simulink model "q3_bilinear"  (R2017b)
settings: Solver=VariableStepAuto  StartTime=0.0  StopTime=5  RelTol=1e-3
settings Model: Creator=admin  LastModifiedBy=admin

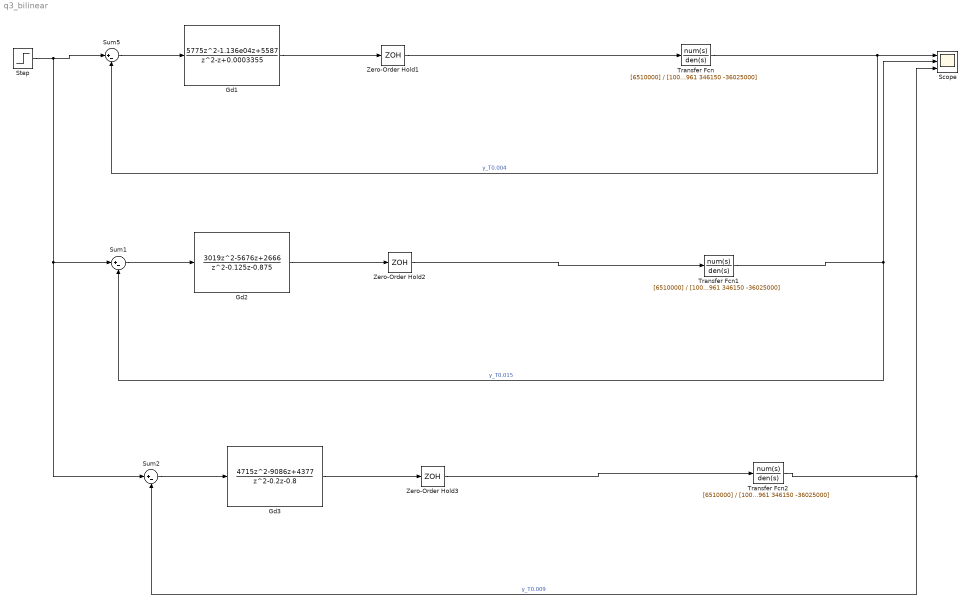
== system q3_bilinear ==
  " Gd1" : DiscreteTransferFcn  Numerator=[5775 -1.136e04 5587]  Denominator=[1 -1 0.0003355]  SampleTime=0.004
  " Gd2" : DiscreteTransferFcn  Numerator=[3019 -5676 2666]  Denominator=[1 -0.125 -0.875]  SampleTime=0.015
  " Gd3" : DiscreteTransferFcn  Numerator=[4715 -9086 4377]  Denominator=[1 -0.2 -0.8]  SampleTime=0.009
  Scope : Scope  NumInputPorts=3
  Step : Step  SampleTime=0
  Sum1 : Sum  Inputs=|+-
  Sum2 : Sum  Inputs=|+-
  Sum5 : Sum  Inputs=|+-
  Transfer Fcn : TransferFcn  Numerator=[6510000]  Denominator=[10000 2501961 346150 -36025000]
  Transfer Fcn1 : TransferFcn  Numerator=[6510000]  Denominator=[10000 2501961 346150 -36025000]
  Transfer Fcn2 : TransferFcn  Numerator=[6510000]  Denominator=[10000 2501961 346150 -36025000]
  Zero-Order Hold1 : ZeroOrderHold  SampleTime=0.004
  Zero-Order Hold2 : ZeroOrderHold  SampleTime=0.015
  Zero-Order Hold3 : ZeroOrderHold  SampleTime=0.00915
  wires:
  Zero-Order Hold2/1 -> Transfer Fcn1/1
  Transfer Fcn1/1 -> Scope/2, Sum1/2  "y_T0.015"
  Transfer Fcn/1 -> Scope/1, Sum5/2  "y_T0.004"
  Transfer Fcn2/1 -> Scope/3, Sum2/2  "y_T0.009"
  " Gd1"/1 -> Zero-Order Hold1/1
  Sum2/1 -> " Gd3"/1
  Zero-Order Hold1/1 -> Transfer Fcn/1
  " Gd3"/1 -> Zero-Order Hold3/1
  Zero-Order Hold3/1 -> Transfer Fcn2/1
  Step/1 -> Sum2/1, Sum1/1, Sum5/1
  Sum1/1 -> " Gd2"/1
  " Gd2"/1 -> Zero-Order Hold2/1
  Sum5/1 -> " Gd1"/1
